simulink model "PID_Contoller"  (R2020b)
settings: Solver=VariableStepAuto  StartTime=0.0  StopTime=10.0  RelTol=1e-3
model mask{Kd=0, Ki=0, Kp=0}
model workspace (MAT data in the model file):
  Kd = 0
  Ki = 0
  Kp = 0
  Ts = Simulink.Parameter
  Ts.Value = 0.01
  Ts.DataType = 'auto'
  Ts.Dimensions = [1 1]
values from neighbouring files (symbols this model uses):
  Ts = 0.01    [Motor_position_data.sldd]
settings Model: ParameterArgumentNames=Kd,Ki,Kp  Creator=Lenovo  LastModifiedBy=Lenovo
settings DataIOCC: SaveOutput=off  SaveTime=off

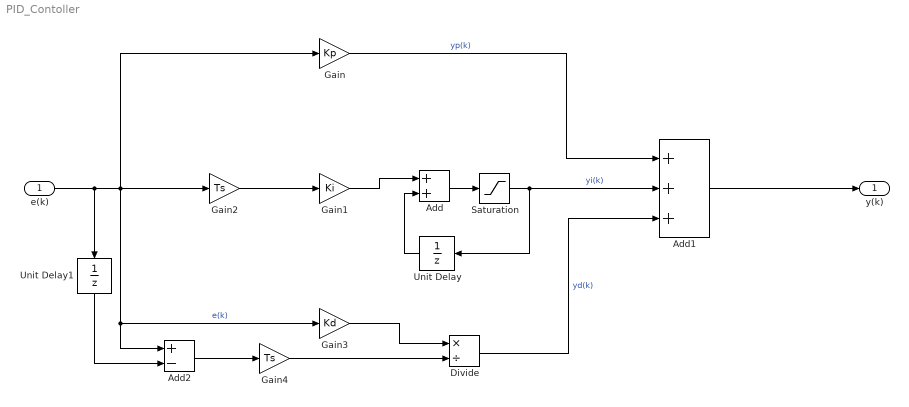
== system PID_Contoller ==
  e(k) : Inport  OutDataTypeStr=double  PortDimensions=1  SampleTime=0
  Add : Sum
  Add1 : Sum  Inputs=+++
  Add2 : Sum  Inputs=+-
  Divide : Product  Inputs=*/
  Gain : Gain  Gain=Kp
  Gain1 : Gain  Gain=Ki
  Gain2 : Gain  Gain=Ts
  Gain3 : Gain  Gain=Kd
  Gain4 : Gain  Gain=Ts
  Saturation : Saturate
  Unit Delay : UnitDelay  SampleTime=-1  HasFrameUpgradeWarning=on
  Unit Delay1 : UnitDelay  SampleTime=-1  HasFrameUpgradeWarning=on
  y(k) : Outport  OutDataTypeStr=double  PortDimensions=1  SampleTime=0
  wires:
  Gain1/1 -> Add/1
  Add/1 -> Saturation/1
  Unit Delay/1 -> Add/2
  Add1/1 -> y(k)/1
  Gain/1 -> Add1/1  "yp(k)"
  Divide/1 -> Add1/3  "yd(k)"
  Unit Delay1/1 -> Add2/2
  e(k)/1 -> Gain/1, Gain3/1, Add2/1, Gain2/1, Unit Delay1/1  "e(k)"
  Add2/1 -> Gain4/1
  Gain4/1 -> Divide/2
  Gain3/1 -> Divide/1
  Gain2/1 -> Gain1/1
  Saturation/1 -> Unit Delay/1, Add1/2  "yi(k)"
